simulink model "SpectrumWirelessChannel_2024b"  (R2024b)
settings: Solver=ode45  StartTime=0.0  StopTime=50000  RelTol=1e-3  EnableMultiTasking=on
PreLoadFcn:
  | c=[1 1 0 0]/sqrt(2);
  | Tf=10000;
  | SNR=25;
  | delta=0.0013;
  | warning off all
undefined symbols (not defined in the file or in its folder): gcbh, rcfiltgaincompat
libraries: commdigbbndpm3 x1, commrandsrc3 x1, commfilt2 x1
settings Model: Creator=morelos_zaragoza  LastModifiedBy=14083
settings SolverCC: AlgebraicLoopSolver=TrustRegion
settings DataIOCC: LimitDataPoints=on  SaveFormat=Array  SignalLoggingSaveFormat=ModelDataLogs  ReturnWorkspaceOutputs=off  SignalLoggingName=sigsOut
settings OptimizationCC: ExpressionDepthLimit=2147483647  InitFltsAndDblsToZero=on  LifeSpan=inf
settings DebuggingCC: AlgebraicLoopMsg=none  SaveWithParameterizedLinksMsg=none  UnderspecifiedInitializationDetection=Classic  MergeDetectMultiDrivingBlocksExec=none  SignalResolutionControl=TryResolveAllWithWarning  MultiTaskDSMMsg=warning  MultiTaskCondExecSysMsg=none  FcnCallInpInsideContextMsg=warning  UnconnectedInputMsg=warning  UnconnectedOutputMsg=warning  UnconnectedLineMsg=warning  StateNameClashWarn=warning  SFUnexpectedBacktrackingDiag=warning  SFNoUnconditionalDefaultTransitionDiag=warning  SFExecutionAtInitializationDiag=none  ArithmeticOperatorsInVariantConditions=warning
settings HardwareCC: ProdBitPerPointer=32  ProdBitPerSizeT=32  ProdBitPerPtrDiffT=32  ProdLargestAtomicFloat=None  ProdIntDivRoundTo=Undefined  ProdEndianess=Unspecified  ProdWordSize=32  ProdHWDeviceType=32-bit Generic  TargetUnknown=on
settings ModelReferenceCC: PropagateSignalLabelsOutOfModel=off
settings SFSimCC: SimUseLocalCustomCode=off  CustomCodeUndefinedFunction=UseInterfaceOnly
settings RTWCC: RTWUseLocalCustomCode=off  GPUComputeCapability=3.5
settings CodeAppCC: StateflowObjectComments=on
settings GRTTargetCC: TargetFcnLib=ansi_tfl_tmw.mat  TargetLangStandard=C89/C90 (ANSI)  CombineOutputUpdateFcns=off  GRTInterface=on
settings ConfigComp: CovMetricSettings=dw  CovSaveCumulativeToWorkspaceVar=on  CovSaveSingleToWorkspaceVar=on  CovExternalEMLEnable=off

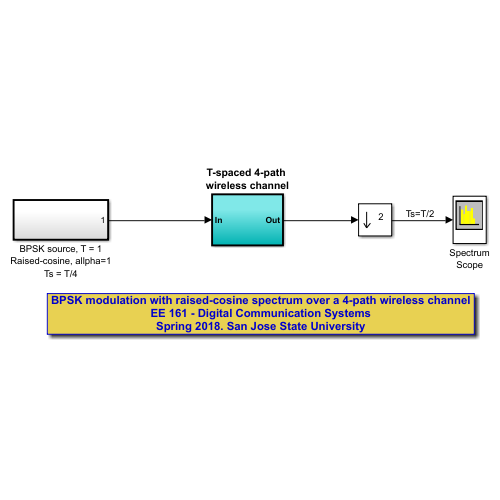
[thumbnail: Simulink's stored preview of the top-level diagram]
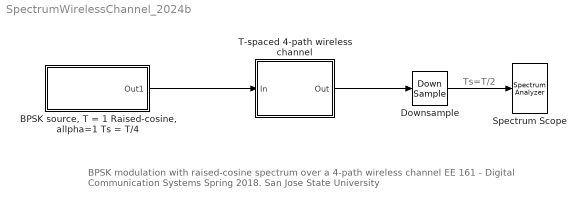
== system SpectrumWirelessChannel_2024b ==
  note: BPSK modulation with raised-cosine spectrum over a 4-path wireless channel
      | EE 161 - Digital Communication Systems
      | Spring 2018. San Jose State University
  note: Ts=T/2
  "BPSK source, T = 1 Raised-cosine, allpha=1 Ts = T/4" : Subsystem  TreatAsAtomicUnit=on
  Downsample : DownSample  RateOptions=Allow multirate processing
  Spectrum Scope : SpectrumAnalyzer  WindowPosition=[738.000000,283.000000,704.000000,500.000000,]  Visible=on  ScopeFrameLocation=window  WindowInvariantSamplesPerUpdate=on  FFTLength=256  YLabel=Magnitude-squared (dBm)  YLimits=[-83.30239415,19.14808979]
  T-spaced 4-path wireless channel : Subsystem  TreatAsAtomicUnit=on
  wires:
  T-spaced 4-path wireless channel/1(Out) -> Downsample/1
  "BPSK source, T = 1 Raised-cosine, allpha=1 Ts = T/4"/1(Out1) -> T-spaced 4-path wireless channel/1(In)
  Downsample/1 -> Spectrum Scope/1

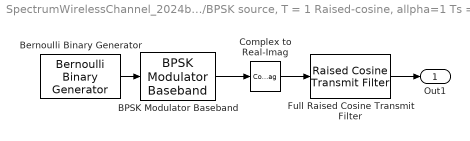
== system SpectrumWirelessChannel_2024b/BPSK source, T = 1 Raised-cosine, allpha=1 Ts = T//4 ==
  BPSK Modulator Baseband : commdigbbndpm3/BPSK Modulator Baseband  Ph=0  outDtype=double  outWordLen=16  outUDDataType=sfix(16)  outFracLenMode=Best precision  outFracLen=15  outDataTypeStr=double  outLastDataTypeStr=double
  Bernoulli Binary Generator : commrandsrc3/Bernoulli Binary Generator  ProbabilityOfZero=0.5  SeedSource=Auto  Seed=0  SampleTime=1  SamplesPerFrame=1  OutputDataType=double  SimulateUsing=Interpreted execution
  Complex to Real-Imag : ComplexToRealImag  Output=Real
  Full Raised Cosine Transmit Filter : commfilt2/Raised Cosine Transmit Filter  filtType=Normal  R=1  filtSpan=2*(4)  N=4  filterGain=rcfiltgaincompat(gcbh)  RateOptions=Allow multirate processing  framing=Allow multirate processing  checkCoeff=off  variableName=rcTxFilt  checkGain=Normalized  sampMode=Mute  saveAsFlag=0  currentFiltSpan=2*(4)  D=4  launchFVT=off  roundingMode=Floor  overflowMode=off  coeffDataTypeStr=Inherit: Same word length as input  coeffMin=[]  coeffMax=[]  coeffLastDataTypeStr=Inherit: Same word length as input  outputDataTypeStr=Inherit: Same as accumulator  outputMin=[]  outputMax=[]  outputLastDataTypeStr=Inherit: Same as accumulator
  Out1 : Outport
  wires:
  Bernoulli Binary Generator/1 -> BPSK Modulator Baseband/1
  BPSK Modulator Baseband/1 -> Complex to Real-Imag/1
  Complex to Real-Imag/1 -> Full Raised Cosine Transmit Filter/1
  Full Raised Cosine Transmit Filter/1 -> Out1/1

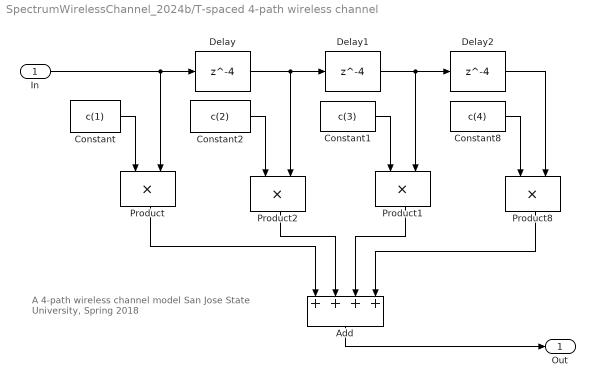
== system SpectrumWirelessChannel_2024b/T-spaced 4-path wireless channel ==
  note: A 4-path wireless channel model
      | San Jose State University, Spring 2018
  In : Inport
  Add : Sum  Inputs=++++
  Constant : Constant  Value=c(1)
  Constant1 : Constant  Value=c(3)
  Constant2 : Constant  Value=c(2)
  Constant8 : Constant  Value=c(4)
  Delay : Delay  DelayLength=4  InitialCondition=0
  Delay1 : Delay  DelayLength=4  InitialCondition=0
  Delay2 : Delay  DelayLength=4  InitialCondition=0
  Product{,1..2,8} (4 alike) : Product  SaturateOnIntegerOverflow=on  OutDataTypeStr=Inherit: Same as first input
  Out : Outport
  wires:
  In/1 -> Product/2, Delay/1
  Delay/1 -> Product2/2, Delay1/1
  Delay2/1 -> Product8/2
  Constant/1 -> Product/1
  Constant8/1 -> Product8/1
  Delay1/1 -> Product1/2, Delay2/1
  Constant1/1 -> Product1/1
  Constant2/1 -> Product2/1
  Add/1 -> Out/1
  Product/1 -> Add/1
  Product2/1 -> Add/2
  Product1/1 -> Add/3
  Product8/1 -> Add/4
